simulink model "M_ZH_Z3"  (R2025a)
settings: Solver=VariableStepAuto  StartTime=0.0  StopTime=2  MaxStep=1e-3  RelTol=1e-3
settings Model: Creator=Szalay  LastModifiedBy=Szalay

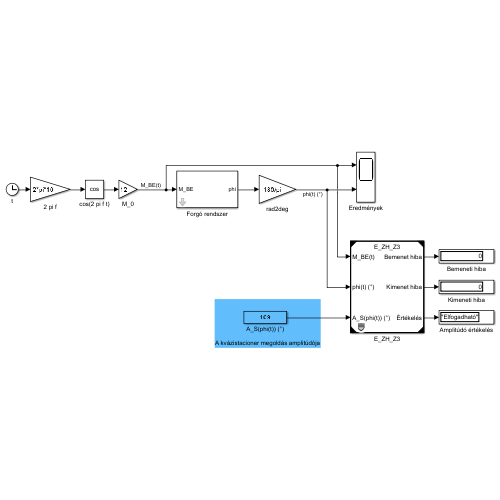
[thumbnail: Simulink's stored preview of the top-level diagram]
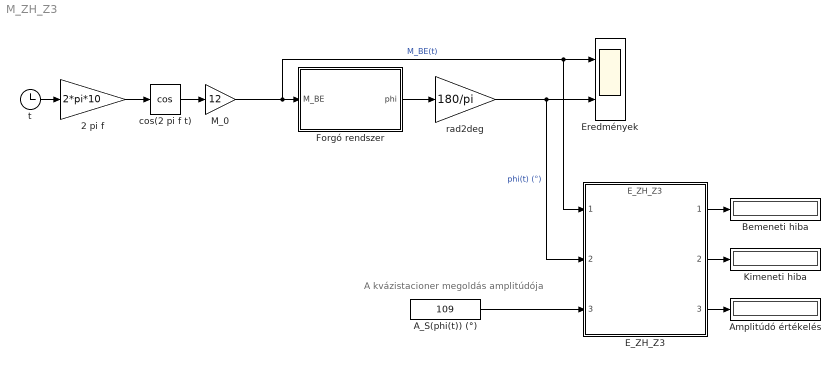
== system M_ZH_Z3 ==
  note: A kvázistacioner megoldás amplitúdója
  2 pi f : Gain  Gain=2*pi*10
  A_S(phi(t)) (°) : Constant  Value=109
  Amplitúdó értékelés : Display
  Bemeneti hiba : Display
  E_ZH_Z3 : ModelReference  ModelNameDialog=E_ZH_Z3.slxp  ModelReferenceVersion=1.15  CopyOfModelProtected=on
  Eredmények : Scope  NumInputPorts=2
      settings: ActiveDisplayYMinimum=-28.685004790156313  ActiveDisplayYMaximum=69.469749949472941
  Forgó rendszer : Subsystem  mask(Forgó rendszer){B=0.1, C=0.5, phi_0=45}
      mask prompts: B "Forgási súrlódási együttható"; C "Csavarási rugómerevség"; phi_0 "Kezdeti szöghelyzet (°)"
      mask DialogControl ParameterGroupVar Prompt: Rendszerparaméter
      mask DialogControl Container3 Prompt: Kezdeti érték
  Kimeneti hiba : Display
  M_0 : Gain  Gain=12
  cos(2 pi f t) : Trigonometry  Operator=cos
  rad2deg : Gain  Gain=180/pi
  t : Clock
  wires:
  rad2deg/1 -> E_ZH_Z3/2, Eredmények/2  "phi(t) (°)"
  M_0/1 -> E_ZH_Z3/1, Eredmények/1, Forgó rendszer/1(M_BE)  "M_BE(t)"
  cos(2 pi f t)/1 -> M_0/1
  2 pi f/1 -> cos(2 pi f t)/1
  t/1 -> 2 pi f/1
  Forgó rendszer/1(phi) -> rad2deg/1
  E_ZH_Z3/1 -> Bemeneti hiba/1
  E_ZH_Z3/2 -> Kimeneti hiba/1
  A_S(phi(t)) (°)/1 -> E_ZH_Z3/3
  E_ZH_Z3/3 -> Amplitúdó értékelés/1

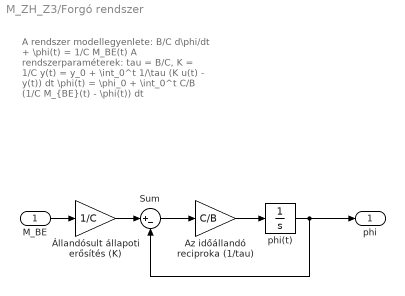
== system M_ZH_Z3/Forgó rendszer ==
  note: A rendszer modellegyenlete:
      |
      | B/C d\phi/dt + \phi(t) = 1/C M_BE(t)
      |
      | A rendszerparaméterek:
      | tau = B/C, K = 1/C
      |
      | y(t) = y_0 + \int_0^t 1/\tau (K u(t) - y(t)) dt
      |
      | \phi(t) = \phi_0 + \int_0^t C/B (1/C M_{BE}(t) - \phi(t)) dt
  M_BE : Inport
  Az időállandó reciproka (1/tau) : Gain  Gain=C/B
  Sum : Sum  Inputs=|+-
  phi(t) : Integrator  InitialCondition=phi_0/180*pi
  Állandósult állapoti erősítés (K) : Gain  Gain=1/C
  phi : Outport
  wires:
  Sum/1 -> Az időállandó reciproka (1/tau)/1
  phi(t)/1 -> phi/1, Sum/2
  Az időállandó reciproka (1/tau)/1 -> phi(t)/1
  Állandósult állapoti erősítés (K)/1 -> Sum/1
  M_BE/1 -> Állandósult állapoti erősítés (K)/1
